simulink model "SchematD1"  (R2015a)
settings: Solver=ode45  SolverMode=SingleTasking  StartTime=0.0  StopTime=10.0  RelTol=1e-3
libraries: simulink_extras x2
settings Model: CovMetricSettings=dwe  CovHtmlReporting=off  covSaveCumulativeToWorkspaceVar=off  CovSaveSingleToWorkspaceVar=off  CovExternalEMLEnable=on  Creator=bartl  LastModifiedBy=bartl
settings DataIOCC: LimitDataPoints=off  SaveFormat=Dataset
settings DebuggingCC: SFUnexpectedBacktrackingDiag=error  SFNoUnconditionalDefaultTransitionDiag=error
settings HardwareCC: ProdBitPerPointer=64  ProdLargestAtomicFloat=Float  ProdIntDivRoundTo=Zero  ProdEndianess=LittleEndian  ProdHWDeviceType=Specified
settings ModelReferenceCC: PropagateSignalLabelsOutOfModel=on
settings SFSimCC: SimUseLocalCustomCode=on
settings RTWCC: RTWUseLocalCustomCode=on
settings GRTTargetCC: TargetLangStandard=C99 (ISO)  GeneratePreprocessorConditionals=Use local settings

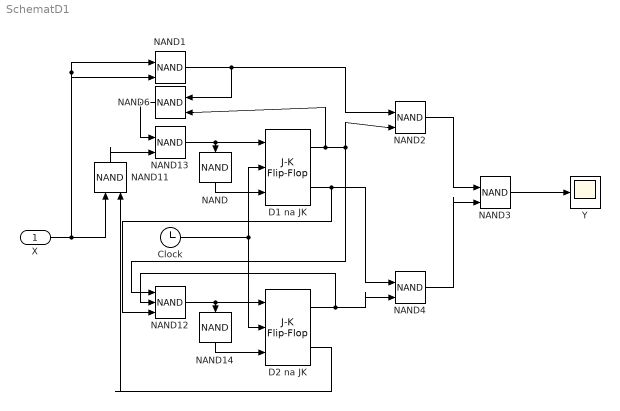
== system SchematD1 ==
  X : Inport
  Clock : Clock
  D1 na JK : simulink_extras/Flip Flops/J-K Flip-Flop  initial_condition=0
  D2 na JK : simulink_extras/Flip Flops/J-K Flip-Flop  initial_condition=0
  NAND : Logic  Operator=NAND  Inputs=1  IconShape=distinctive  AllPortsSameDT=off  OutDataTypeStr=boolean
  NAND{1..4,6,11,13} (7 alike) : Logic  Operator=NAND  IconShape=distinctive  AllPortsSameDT=off  OutDataTypeStr=boolean
  NAND12 : Logic  Operator=NAND  Inputs=3  IconShape=distinctive  AllPortsSameDT=off  OutDataTypeStr=boolean
  NAND14 : Logic  Operator=NAND  Inputs=1  IconShape=distinctive  AllPortsSameDT=off  OutDataTypeStr=boolean
  Y : Scope
      settings: TimeRange=auto  MaxDataPoints=5000  SaveToWorkspace=off  SaveName=ScopeData  YMin=-10  YMax=10  SampleTime=-1
  wires:
  NAND/1 -> D1 na JK/3
  NAND14/1 -> D2 na JK/3
  NAND13/1 -> NAND/1, D1 na JK/1
  NAND12/1 -> NAND14/1, D2 na JK/1
  Clock/1 -> D2 na JK/2, D1 na JK/2
  X/1 -> NAND11/1, NAND1/2, NAND1/1
  D1 na JK/1 -> NAND6/2, NAND12/1, NAND2/2
  NAND1/1 -> NAND6/1, NAND2/1
  D2 na JK/1 -> NAND12/2, NAND4/2
  D1 na JK/2 -> NAND12/3, NAND4/1
  NAND2/1 -> NAND3/1
  NAND4/1 -> NAND3/2
  NAND3/1 -> Y/1
  NAND6/1 -> NAND13/1
  NAND11/1 -> NAND13/2
  D2 na JK/2 -> NAND11/2
